simulink model "EMD_model_2"  (R2019a)
settings: Solver=ode45  StartTime=0  StopTime=setStopTime  FixedStep=0.0005  RelTol=1e-3  EnableMultiTasking=on
model workspace (MAT data in the model file):
  MCOS : class17 (value not decoded)
  MCOS : class17 (value not decoded)
  MCOS : class17 (value not decoded)
  bodyAmp = 0
  bodyPhase = 0
  freq = 0.628318530718
  headAmp = 0
  headPhase = 0
  high_delay = 0
  imageData = [0.00228480667088 0.00685422825671 0.0114230745906 0.0159909622235 0.0205575077854 0.0251223280162 0.0296850397975 0.0342452601838 0.0388026064343 0.0433566960441 0.0479071467754 0.0524535766893 ... (8204 elements, 1x8204)]
  low_delay = 0.035
  outputTimeList = [10 10.1 10.2 10.3 10.4 10.5 10.6 10.7 10.8 10.9 11 11.1 ... (101 elements, 101x1)]
  photo_a = [1 280.74949398 32070.4687612 642041.021699]
  photo_b = [0 0 0 1204751481.42]
  setStartTime = 5.68986602902
  setStopTime = 20
  stimAmp = 15
  temporalFilt = 0.035
  timeConstant = 0.06
libraries: visionsources x1
(part 2 of 2)

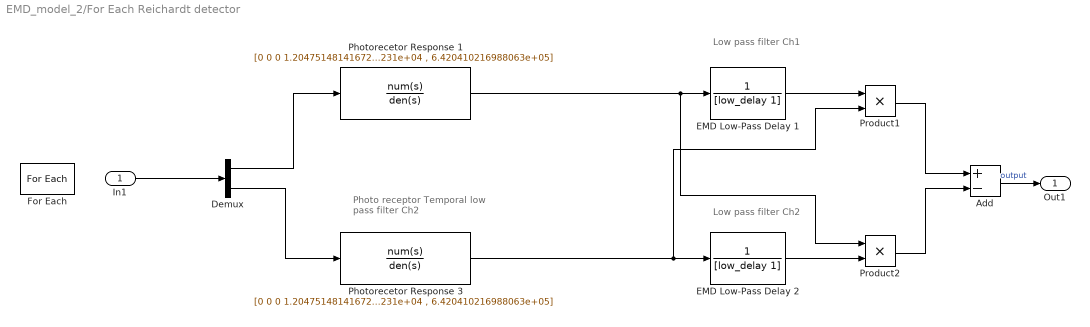
== system EMD_model_2/For Each Reichardt detector ==
  note: Photo receptor
      | Temporal low pass filter
      | Ch2
  note: Low pass filter
      | Ch1
  note: Low pass filter
      | Ch2
  In1 : Inport  Partition=on  PartitionDimension=1  PartitionWidth=1  PartitionOffset=0
  Add : Sum  Inputs=+-
  Demux : Demux  Outputs=2
  EMD Low-Pass Delay 1 : TransferFcn  Denominator=[low_delay 1]
  EMD Low-Pass Delay 2 : TransferFcn  Denominator=[low_delay 1]
  For Each : ForEach  DisableCoverage=on  IndexMode=One-based
  Photorecetor Response 1 : TransferFcn  Numerator=[0 0 0 1.204751481416720e+09]  Denominator=[1 , 2.807494939800572e+02 , 3.207046876121231e+04 , 6.420410216988063e+05]
  Photorecetor Response 3 : TransferFcn  Numerator=[0 0 0 1.204751481416720e+09]  Denominator=[1 , 2.807494939800572e+02 , 3.207046876121231e+04 , 6.420410216988063e+05]
  Product1 : Product  RndMeth=Zero
  Product2 : Product  RndMeth=Zero
  Out1 : Outport  ConcatenationDimension=1
  wires:
  EMD Low-Pass Delay 1/1 -> Product1/1
  Product1/1 -> Add/1
  Product2/1 -> Add/2
  EMD Low-Pass Delay 2/1 -> Product2/2
  Add/1 -> Out1/1  "output"
  In1/1 -> Demux/1
  Demux/1 -> Photorecetor Response 1/1
  Demux/2 -> Photorecetor Response 3/1
  Photorecetor Response 1/1 -> EMD Low-Pass Delay 1/1, Product2/1
  Photorecetor Response 3/1 -> EMD Low-Pass Delay 2/1, Product1/2

== matlab function EMD_model_2/sampleImage ==
  data: imageData input; intensity output double size=360,2; seenAngle input
function intensity = fcn(imageData,seenAngle)
%#codegen

imageWidth = length(imageData);

% Subsample with resolution of compound eye
sampleCoord = 0:359;
sampleCoord = sampleCoord + seenAngle;
sampleCoord = mod(sampleCoord,360);
temp        = interp1(linspace(0,360,imageWidth),imageData,sampleCoord);

% Create output signals
intensity = [temp(:), circshift(temp(:),-1)];
